simulink model "ConfigurableSubsystem"  (R2015b)
settings: Solver=VariableStepAuto  StartTime=0.0  StopTime=10.0  RelTol=1e-3
libraries: LibConfigurableSubsystem x1
settings Model: Creator=LUBO  LastModifiedBy=LUBO

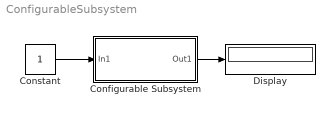
== system ConfigurableSubsystem ==
  Configurable Subsystem : Subsystem  BlockChoice=Subsystem1
      settings: AttributesFormatString=%<BlockChoice>  MemberBlocks=Subsystem,Subsystem1,Subsystem2
      settings: TemplateBlock=|
      | LibConfigurableSubsystem/Configurable
      | Subsystem
  Constant : Constant
  Display : Display
  wires:
  Configurable Subsystem/1(Out1) -> Display/1
  Constant/1 -> Configurable Subsystem/1(In1)

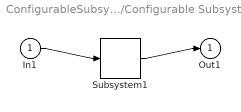
== system ConfigurableSubsystem/Configurable Subsystem ==
  In1 : Inport
  Subsystem1 : LibConfigurableSubsystem/Subsystem1
  Out1 : Outport
  wires:
  In1/1 -> Subsystem1/1
  Subsystem1/1 -> Out1/1
